simulink model "Chopper"  (R2022a)
settings: Solver=VariableStepAuto  StartTime=0.0  StopTime=1  RelTol=1e-3
libraries: spsMeanLib x6, spsDCVoltageSourceLib x2, spsDiodeLib x2, spsIGBTLib x2, spsDCMachineLib x1, spsVoltageMeasurementLib x1, spspowerguiLib x1
settings Model: Creator=ASUTOSH MISHRA  LastModifiedBy=ASUTOSH MISHRA
settings SolverCC: ZeroCrossAlgorithm=Adaptive
settings DebuggingCC: IgnoredZcDiagnostic=none

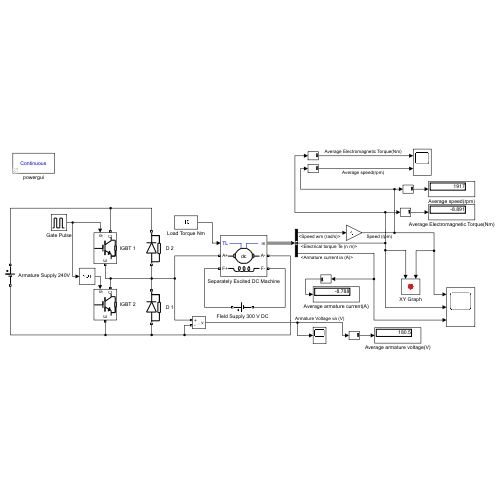
[thumbnail: Simulink's stored preview of the top-level diagram]
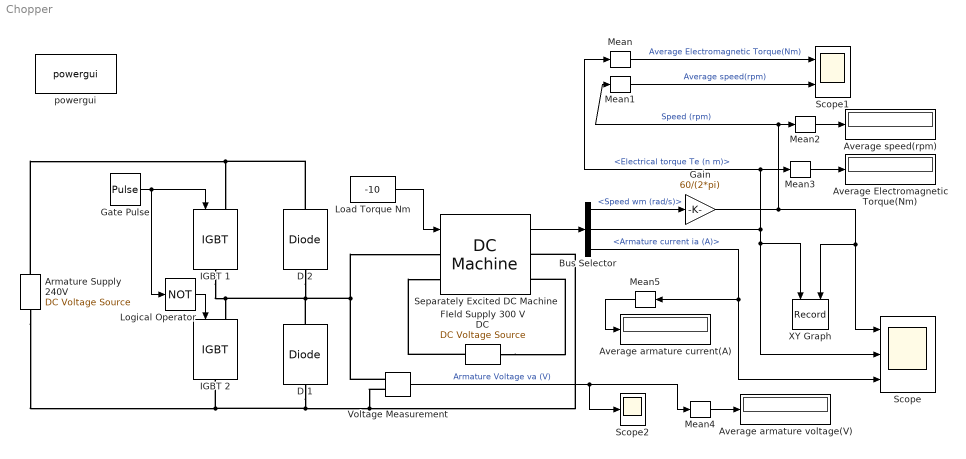
== system Chopper ==
  Armature Supply 240V : spsDCVoltageSourceLib/DC Voltage Source  Amplitude=240  Measurements=None
  Average Electromagnetic Torque(Nm) : Display
  Average armature current(A) : Display
  Average armature voltage(V) : Display
  Average speed(rpm) : Display
  Bus Selector : BusSelector  OutputSignals=Speed wm (rad/s),Electrical torque Te (n m),Armature current ia (A)
  D 1 : spsDiodeLib/Diode  Ron=0.001  Lon=0  Vf=0.8  IC=0  UseSnubber=0  Rs=500  Cs=250e-9  Measurements=off
  D 2 : spsDiodeLib/Diode  Ron=0.001  Lon=0  Vf=0.8  IC=0  UseSnubber=0  Rs=500  Cs=250e-9  Measurements=off
  FIeld Supply 300 V DC : spsDCVoltageSourceLib/DC Voltage Source  Amplitude=300  Measurements=None
  Gain : Gain  Gain=60/(2*pi)
  Gate Pulse : DiscretePulseGenerator  PulseType=Time based  Amplitude=10  Period=.02  PulseWidth=75
  IGBT 1 : spsIGBTLib/IGBT  Ron=0.001  Lon=0  Vf=1  Tf=1e-6  Tt=2e-6  IC=0  Rs=1e5  Cs=inf  Measurements=off
  IGBT 2 : spsIGBTLib/IGBT  Ron=0.001  Lon=0  Vf=1  Tf=1e-6  Tt=2e-6  IC=0  Rs=1e5  Cs=inf  Measurements=off
  Load Torque Nm : Constant  Value=-10
  Logical Operator : Logic  Operator=NOT  Inputs=1  AllPortsSameDT=off  OutDataTypeStr=boolean
  Mean{,1..5} (6 alike) : spsMeanLib/Mean  Freq=50  Vinit=0  Ts=0
  Scope : Scope  NumInputPorts=3
  Scope1 : Scope  NumInputPorts=2
  Scope2 : Scope
  Separately Excited DC Machine : spsDCMachineLib/DC Machine  PresetModel=01: 5HP 240V 1750RPM Field:300V  MechanicalLoad=Torque TL  FieldType=Wound  ShowDetailedParameters=on  MeasurementBus=off  RLa=[2.581 0.028]  RLf=[281.2 156]  Laf=0.9483  MachineConstant=Torque constant (N.m/A)  Ke=1.8  Kt=1.8  J=0.02215  Bm=0.002953  Tf=0.5161  w0=0  Ifinit=1.06685633001422  TsPowergui=0  TsBlock=-1
  Voltage Measurement : spsVoltageMeasurementLib/Voltage Measurement  PhasorSimulation=off  OutputType=Complex  PSBequivalent=0
  XY Graph : Record  FileSettingsInternal="{\"entries\":[{\"content\":{\"excelSettings\":{\"content\":{},\"type\":\"Streamout.ExcelSettings\"}},\"type\":\"Streamout.FileSettingStorage\",\"uuid\":\"\"}],\"packageUris\":[\"http:\\/\\/schema.mathworks.com\\/mf0\\/streamout_blocks\\/R2020a\"],\"version\":\"1.0\"}"  Layout=[1 1]  SignalsInternal="{\"entries\":[{\"content\":{\"signals\":[{\"content\":{\"blockPath\":[],\"channel\":[],\"dimensions\":[1],\"domain\":\"\",\"lineColor\":\"#a2142f\",\"plots\":[1],\"port\":1,\"sid\":[\"\"],\"signalID\":4242,\"signalName\":\"<Electrical torque Te (n m)>\"},\"type\":\"RecordBlkView.Signal\",\"uuid\":\"\"},{\"content\":{\"blockPath\":[],\"channel\":[],\"dimensions\":[1],\"domain\":\"\",\"lineColor\":\"#139fff\",\"plots\":[1],\"port\":2,\"sid\":[\"\"],\"signalID\":4246,\"signalName\":\"Speed (rpm)\"},\"type\":\"RecordBlkView.Signal\",\"uuid\":\"\"}]},\"type\":\"RecordBlkView.InputSignals\",\"uuid\":\"\"}],\"packageUris\":[\"http:\\/\\/schema.mathworks.com\\/mf0\\/streamout_blocks\\/R2020a\"],\"version\":\"1.0\"}"  VisualizationBindings="{\"xyplotplugin\":{\"info\":[{\"series\":[{\"bindingParametersList\":[{\"parameter\":\"X-Axis\",\"signalID\":4242,\"signalName\":\"<Electrical torque Te (n m)>\"},{\"parameter\":\"Y-Axis\",\"signalID\":4246,\"signalName\":\"Speed (rpm)\"}],\"seriesID\":6805}],\"subplotID\":1}]}}"  CompatibilityTag=XY
  powergui : spspowerguiLib/powergui  Priority=1  SimulationMode=Continuous  SampleTime=.0002  frequency=60  Iterations=50  frequencyindice=0  Pbase=100e6  ErrMax=1e-4  UnitsV=kV  UnitsW=MW  buscounter=0  FunctionMessages=off  echomessages=off  EnableUseOfTLC=off  CurrentSourceSwitches=off  DisableSnubberDevices=off  DisableRonSwitches=off  DisableVfSwitches=off  DisplayEquations=off  AutomaticDiscreteSolvers=off  SolverType=Tustin/Backward Euler (TBE)  Interpol=off  ExternalGateDelay=off  methode=off  Ts=100  x0status=blocks  SPID=on  SwTol=0  HookPort=off  NonlinearTolerance=1e-4  nMaxIteration=100  ContinueOnMaxIteration=off  RestoreLinks=warning  ResistiveCurrentMeasurement=off  Frange=[0:2:500]  Ylog=off  Xlog=on  ShowGrid=off  save=off  variable=ZData  structure=0  ZoomFFT=off  StartTime=0.0  cycles=1  DisplayStyle=1  fundamental=60  FreqAxis=off  MaxFrequency=1000  frequencyindicesteady=1  RmsSteady=1  display=off
  wires:
  Separately Excited DC Machine/1 -> Bus Selector/1
  Bus Selector/1 -> Gain/1  "<Speed wm (rad/s)>"
  Bus Selector/2 -> XY Graph/1, Scope/2, Mean3/1, Mean/1  "<Electrical torque Te (n m)>"
  Gate Pulse/1 -> Logical Operator/1, IGBT 1/1
  Logical Operator/1 -> IGBT 2/1
  Voltage Measurement/1 -> Scope2/1, Mean4/1  "Armature Voltage va (V)"
  Bus Selector/3 -> Mean5/1, Scope/3  "<Armature current ia (A)>"
  Mean1/1 -> Scope1/2  "Average speed(rpm)"
  Mean/1 -> Scope1/1  "Average Electromagnetic Torque(Nm)"
  Mean2/1 -> Average speed(rpm)/1
  Mean3/1 -> Average Electromagnetic Torque(Nm)/1
  Gain/1 -> XY Graph/2, Scope/1, Mean1/1, Mean2/1  "Speed (rpm)"
  Mean4/1 -> Average armature voltage(V)/1
  Mean5/1 -> Average armature current(A)/1
  Load Torque Nm/1 -> Separately Excited DC Machine/1
  connections:
  Armature Supply 240V/RConn1 -- D 2/RConn1 -- IGBT 1/LConn1
  Armature Supply 240V/LConn1 -- D 1/LConn1 -- Separately Excited DC Machine/RConn1 -- Voltage Measurement/LConn2 -- IGBT 2/RConn1
  FIeld Supply 300 V DC/RConn1 -- Separately Excited DC Machine/LConn2
  FIeld Supply 300 V DC/LConn1 -- Separately Excited DC Machine/RConn2
  D 2/LConn1 -- Separately Excited DC Machine/LConn1 -- Voltage Measurement/LConn1 -- D 1/RConn1 -- IGBT 2/LConn1 -- IGBT 1/RConn1
